simulink model "tank3"  (R2020b)
settings: Solver=VariableStepAuto  StartTime=0.0  StopTime=40000  RelTol=1e-3
values from neighbouring files (symbols this model uses):
  a_out = 0    [TankFillingScript.m]
  c = 16    [TankFillingScript.m]
  k_out = 0.1587/60    (= 0.002645)    [TankFillingScript.m]
settings Model: Creator=StevensUser  LastModifiedBy=mreiff

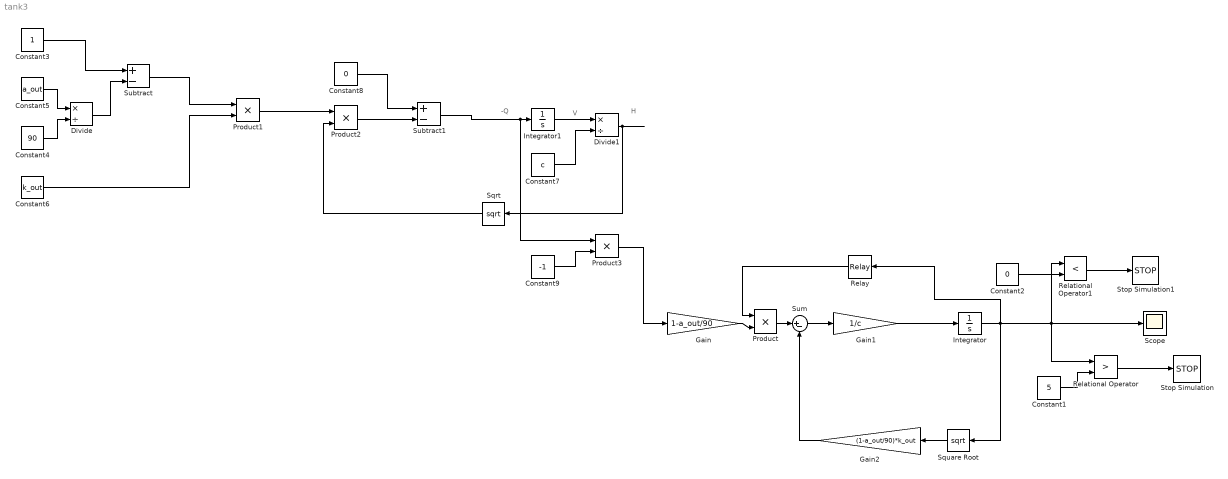
== system tank3 ==
  note: -Q
  note: V
  note: H
  Constant1 : Constant  Value=5
  Constant2 : Constant  Value=0
  Constant3 : Constant
  Constant4 : Constant  Value=90
  Constant5 : Constant  Value=a_out
  Constant6 : Constant  Value=k_out
  Constant7 : Constant  Value=c
  Constant8 : Constant  Value=0
  Constant9 : Constant  Value=-1
  Divide : Product  Inputs=*/
  Divide1 : Product  Inputs=*/
  Gain : Gain  Gain=1-a_out/90
  Gain1 : Gain  Gain=1/c
  Gain2 : Gain  Gain=(1-a_out/90)*k_out
  Integrator : Integrator
  Integrator1 : Integrator  InitialCondition=64
  Product{,1..3} (4 alike) : Product
  Relational Operator : RelationalOperator  Operator=>  OutDataTypeStr=boolean  RndMeth=Simplest
  Relational Operator1 : RelationalOperator  Operator=<  OutDataTypeStr=boolean  RndMeth=Simplest
  Relay : Relay  OnSwitchValue=4.1  OffSwitchValue=3.9  OnOutputValue=0  OffOutputValue=1
  Scope : Scope
  Sqrt : Sqrt  SaturateOnIntegerOverflow=on
  Square Root : Sqrt  SaturateOnIntegerOverflow=on
  Stop Simulation : Stop
  Stop Simulation1 : Stop
  Subtract : Sum  Inputs=+-
  Subtract1 : Sum  Inputs=+-
  Sum : Sum  Inputs=|+-
  wires:
  Product3/1 -> Gain/1
  Gain1/1 -> Integrator/1
  Relational Operator/1 -> Stop Simulation/1
  Constant1/1 -> Relational Operator/2
  Sum/1 -> Gain1/1
  Gain2/1 -> Sum/2
  Square Root/1 -> Gain2/1
  Constant2/1 -> Relational Operator1/2
  Relational Operator1/1 -> Stop Simulation1/1
  Gain/1 -> Product/2
  Product/1 -> Sum/1
  Integrator/1 -> Square Root/1, Relational Operator/1, Scope/1, Relational Operator1/1, Relay/1
  Relay/1 -> Product/1
  Subtract1/1 -> Product3/1, Integrator1/1
  Constant6/1 -> Product1/2
  Subtract/1 -> Product1/1
  Product2/1 -> Subtract1/2
  Sqrt/1 -> Product2/2
  Constant8/1 -> Subtract1/1
  Divide1/1 -> Sqrt/1
  Constant7/1 -> Divide1/2
  Constant4/1 -> Divide/2
  Constant3/1 -> Subtract/1
  Integrator1/1 -> Divide1/1
  Constant5/1 -> Divide/1
  Divide/1 -> Subtract/2
  Product1/1 -> Product2/1
  Constant9/1 -> Product3/2
